simulink model "ModularSIM3D"  (R2023b)
settings: Solver=VariableStepAuto  StartTime=0.0  StopTime=10.0  RelTol=1e-3
libraries: vrlib x1
settings Model: Creator=arnaud  LastModifiedBy=isido

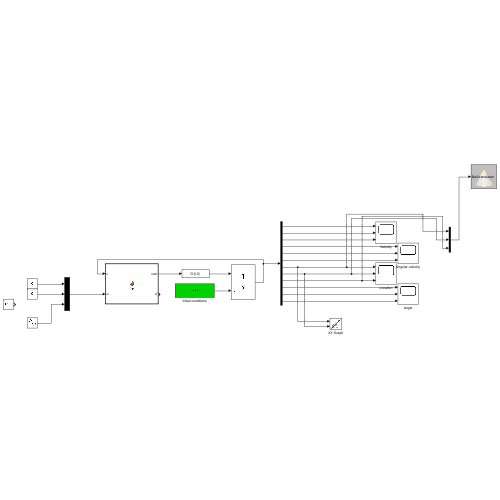
[thumbnail: Simulink's stored preview of the top-level diagram]
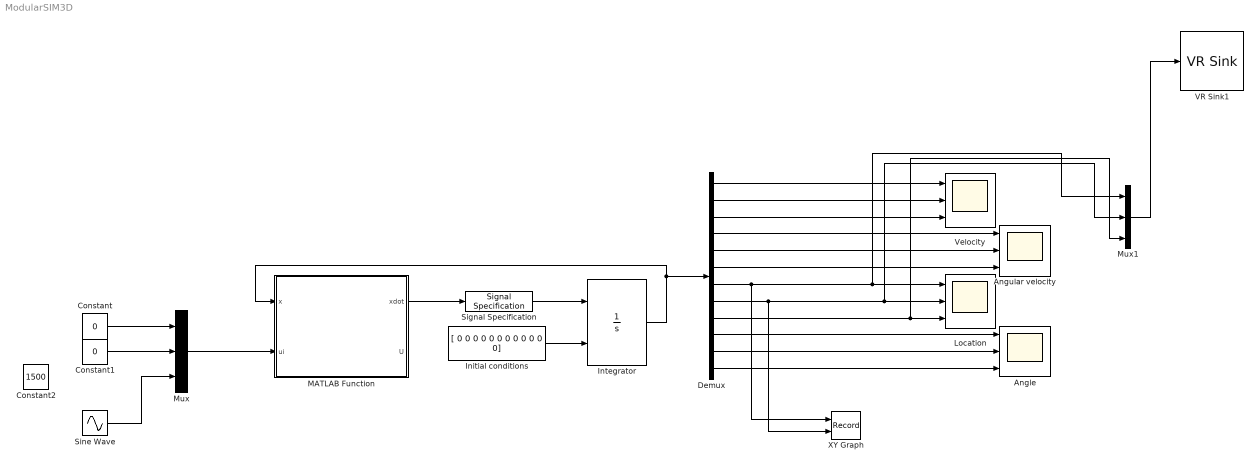
== system ModularSIM3D ==
  Angle : Scope  NumInputPorts=3
  Angular velocity : Scope  NumInputPorts=3
  Constant : Constant  Value=0
  Constant1 : Constant  Value=0
  Constant2 : Constant  Value=1500
  Demux : Demux  Outputs=12
  Initial conditions : Constant  Value="[ 0 0 0 0 0 0 0 0  0 0 0 0]"
  Integrator : Integrator  InitialConditionSource=external  InitialCondition=zeros(1,12)'
  Location : Scope  NumInputPorts=3
  MATLAB Function : MATLAB Function  TreatAsAtomicUnit=on
  Mux : Mux  Inputs=3
  Mux1 : Mux  Inputs=3
  Signal Specification : SignalSpecification  Dimensions=[12]
  Sine Wave : Sin  Amplitude=1500  SampleTime=0
  VR Sink1 : vrlib/VR Sink  InstantiateOnLoad=on  SampleTime=0.1  ViewEnable=on  RemoteChange=off  RemoteView=off  FieldsWritten=Ball.translation.3.1.1.double  WorldFileName=ball_test.x3d  AutoView=off  VideoDimensions=[]  AllowVariableSize=off
  Velocity : Scope  NumInputPorts=3
  XY Graph : Record  FileSettingsInternal="{\"entries\":[{\"content\":{\"excelSettings\":{\"content\":{},\"type\":\"Streamout.ExcelSettings\"}},\"type\":\"Streamout.FileSettingStorage\",\"uuid\":\"\"}],\"packageUris\":[\"http:\\/\\/schema.mathworks.com\\/mf0\\/streamout_blocks\\/R2020a\"],\"version\":\"1.0\"}"  Layout=[1 1]  SignalsInternal="{\"entries\":[{\"content\":{\"signals\":[{\"content\":{\"blockPath\":[],\"dimensions\":[1],\"domain\":\"\",\"lineColor\":\"#0072bd\",\"port\":1,\"sid\":[\"\"],\"signalID\":134,\"signalName\":\"Demux:7\"},\"type\":\"RecordBlkView.Signal\",\"uuid\":\"\"},{\"content\":{\"blockPath\":[],\"dimensions\":[1],\"domain\":\"\",\"lineColor\":\"#d95319\",\"port\":2,\"sid\":[\"\"],\"signalID\":138,\"signalName\":\"Demux:8\"},\"type\":\"RecordBlkView.Signal\",\"uuid\":\"\"}]},\"type\":\"RecordBlkView.InputSignals\",\"uuid\":\"\"}],\"packageUris\":[\"http:\\/\\/schema.mathworks.com\\/mf0\\/streamout_blocks\\/R2020a\"],\"version\":\"1.0\"}"  VisualizationBindings="{\"xyplotplugin\":{\"info\":[{\"series\":[],\"subplotID\":1}]}}"  CompatibilityTag=XY
  wires:
  Mux/1 -> MATLAB Function/2(ui)
  Constant1/1 -> Mux/2
  Constant/1 -> Mux/1
  Initial conditions/1 -> Integrator/2
  Integrator/1 -> MATLAB Function/1(x), Demux/1
  MATLAB Function/1(xdot) -> Signal Specification/1
  Signal Specification/1 -> Integrator/1
  Demux/1 -> Velocity/1
  Demux/7 -> XY Graph/1, Mux1/1, Location/1
  Demux/6 -> Angular velocity/3
  Demux/4 -> Angular velocity/1
  Demux/5 -> Angular velocity/2
  Demux/8 -> XY Graph/2, Mux1/2, Location/2
  Demux/9 -> Mux1/3, Location/3
  Demux/2 -> Velocity/2
  Demux/3 -> Velocity/3
  Demux/10 -> Angle/1
  Demux/11 -> Angle/2
  Demux/12 -> Angle/3
  Mux1/1 -> VR Sink1/1
  Sine Wave/1 -> Mux/3

== matlab function ModularSIM3D/MATLAB Function ==
  data: x input; xdot output size=12; ui input; U output
function [xdot,U] = fcn(x,ui)

[xdot,U] = main_Modular(x,ui);
